simulink model "prova2"  (R2024a)
settings: Solver=ode23t  StartTime=0.0  StopTime=simT  RelTol=1e-3  AbsTol=1e-3
PreLoadFcn:
  | sscv_wind_turbine_input
undefined symbols (not defined in the file): actuatorRampRate, brakePressure, controllerTimeConstant, Derating, ee_sli_rtmsupport, G, gcbh, generatorEfficiency, generatorLumpedInductance, generatorLumpedResistance, gridFrequency, iGenerationGain, maxPitchAngle, minPitchAngle, mpptOmega, mpptPower, mpptWindSpeed, pGenerationGain, pGeneratorBrakeLimit, pitchBrakeAngle, turbineRatedPower, vWindRated, wAtGeneratorRatedPower, wGeneratorBrakeLimit
libraries: fl_lib x19, simulink x15, nesl_utility x14, ee_lib x10, sdl_lib x6, eeGeneralControl x3, eeGeneralMeasurement x2
(part 2 of 2)

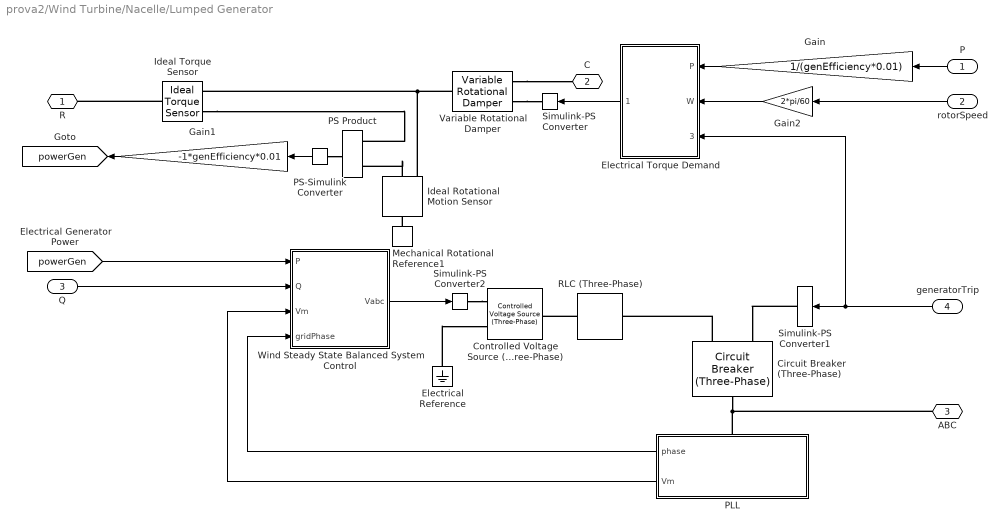
== system prova2/Wind Turbine/Nacelle/Lumped Generator ==
  P : Inport
  rotorSpeed : Inport  Port=2
  Q : Inport  Port=3
  generatorTrip : Inport  Port=4
  Circuit Breaker (Three-Phase) : ee_lib/Switches & Breakers/Circuit Breaker (Three-Phase)  R_closed=1e-5 Ohm  G_open=1e-8 1/Ohm  threshold=0.5 V  breaker_behavior=ee.enum.switches.breakerBehavior.zeroCrossingEnable
      settings: InternalSimscapePortConfiguration="{\"Bottom\":[],\"Left\":[{\"id\":\"vT\",\"label\":\"vT\",\"type\":\"input\"},{\"id\":\"N1\",\"label\":\"~1\",\"type\":\"foundation.electrical.three_phase\"}],\"Right\":[{\"id\":\"N2\",\"label\":\"~2\",\"type\":\"foundation.electrical.three_phase\"}],\"Top\":[]}"
  Controlled Voltage Source (Three-Phase) : ee_lib/Sources/Controlled Voltage Source (Three-Phase)  input_option=ee.enum.inputType.instantaneous  FRated=60 Hz
      settings: InternalSimscapePortConfiguration="{\"Bottom\":[],\"Left\":[{\"id\":\"S\",\"label\":\"S\",\"type\":\"input\"},{\"id\":\"n\",\"label\":\"n\",\"type\":\"foundation.electrical.electrical\"}],\"Right\":[{\"id\":\"N\",\"label\":\"~\",\"type\":\"foundation.electrical.three_phase\"}],\"Top\":[]}"
  Electrical Reference : fl_lib/Electrical/Electrical Elements/Electrical Reference
  Electrical Torque Demand : Subsystem
  Gain : Gain  Gain=1/(genEfficiency*0.01)
  Gain1 : Gain  Gain=-1*genEfficiency*0.01
  Gain2 : Gain  Gain=2*pi/60
  Ideal Rotational Motion Sensor : fl_lib/Mechanical/Mechanical Sensors/Ideal Rotational Motion Sensor  reference=foundation.enum.MeasurementReference.difference  acceleration_port=false  velocity_port=true  position_port=true  wrap_angle=simscape.enum.onoff.off  offset=0 rad
  Ideal Torque Sensor : fl_lib/Mechanical/Mechanical Sensors/Ideal Torque Sensor
  Mechanical Rotational Reference1 : fl_lib/Mechanical/Rotational Elements/Mechanical Rotational Reference
  PLL : Subsystem
      settings: PortSchema="{\"entries\":[{\"content\":{\"sides\":[{\"content\":{\"connectorIds\":[\"LConn1\"]},\"type\":\"ConnectorPlacement.EquallySpacedRectSide\",\"uuid\":\"d52864e1-db35-4dad-add5-1ee067043f1c\"},{\"content\":{\"connectorIds\":[],\"side\":\"RIGHT\"},\"type\":\"ConnectorPlacement.EquallySpacedRectSide\",\"uuid\":\"a5ba0e67-56ea-44cb-9ec3-4038d29660fe\"},{\"content\":{\"connectorIds\":[],\"side\":\"TOP\"},\"type\":\"ConnectorPlacement.EquallySpacedRectSide\",\"uuid\":\"5a398043-7e81-49e7-beae-eacc9cf31df4\"},{\"content\":{\"connectorIds\":[\"Out1\",\"Out2\"],\"side\":\"BOTTOM\"},\"type\":\"ConnectorPlacement.EquallySpacedRectSide\",\"uuid\":\"36c29948-68bf-4126-b9d0-685ba9cc8aca\"}]},\"type\":\"ConnectorPlacement.EquallySpacedConnector\",\"uuid\":\"348acdbb-59d7-41c8-861d-aa801afd2b04\"}],\"packageUris\":[\"http://schema.mathworks.com/mf0/Connector/R2020b\"],\"version\":\"1.0\"}"
  PS Product : fl_lib/Physical Signals/Functions/PS Product
  PS-Simulink Converter : nesl_utility/PS-Simulink Converter  PhysicalDomain=network_engine_domain  SubClassName=ps_output  LeftPortType=input  RightPortType=output  PseudoPeriodic=off  Frequencies=[]  VectorFormat=inherit  Unit=inherit  AffineConversion=off
  RLC (Three-Phase) : ee_lib/Passive/RLC Assemblies/RLC (Three-Phase)  component_structure=ee.enum.rlc.structure.SeriesRL  R=genResistor Ohm  L=genInductance H  C=1e-6 F  R_parasitic=0 Ohm  G_parasitic=0 1/Ohm  IL_specify=off  IL_priority=High  IL=[0, 0, 0] A  IL_nominal_specify=off  IL_nominal_value=1  IL_nominal_unit=A  VC_specify=off  VC_priority=High  VC=[0, 0, 0] V  VC_nominal_specify=off  VC_nominal_value=1  VC_nominal_unit=V
      settings: InternalSimscapePortConfiguration="{\"Bottom\":[],\"Left\":[{\"id\":\"N1\",\"label\":\"~1\",\"type\":\"foundation.electrical.three_phase\"}],\"Right\":[{\"id\":\"N2\",\"label\":\"~2\",\"type\":\"foundation.electrical.three_phase\"}],\"Top\":[]}"
  Simulink-PS Converter : nesl_utility/Simulink-PS Converter  PhysicalDomain=network_engine_domain  SubClassName=ps_input  LeftPortType=input  RightPortType=output  PseudoPeriodic=off  Frequencies=[]  NoiseDistribution=none  NoiseParameters=[]  Unit=N*m/(rad/s)  AffineConversion=off  FilteringAndDerivatives=provide  SimscapeFilterOrder=1  InputFilterTimeConstant=0.001  UdotUserProvided=0
  Simulink-PS Converter1 : nesl_utility/Simulink-PS Converter  PhysicalDomain=network_engine_domain  SubClassName=ps_input  LeftPortType=input  RightPortType=output  PseudoPeriodic=off  Frequencies=[]  NoiseDistribution=none  NoiseParameters=[]  Unit=V  AffineConversion=off  FilteringAndDerivatives=provide  SimscapeFilterOrder=1  InputFilterTimeConstant=0.001  UdotUserProvided=0
  Simulink-PS Converter2 : nesl_utility/Simulink-PS Converter  PhysicalDomain=network_engine_domain  SubClassName=ps_input  LeftPortType=input  RightPortType=output  PseudoPeriodic=off  Frequencies=[]  NoiseDistribution=none  NoiseParameters=[]  Unit=V  AffineConversion=off  FilteringAndDerivatives=provide  SimscapeFilterOrder=1  InputFilterTimeConstant=0.001  UdotUserProvided=0
  Variable Rotational Damper : sdl_lib/Couplings & Drives/Springs & Dampers/Variable Rotational Damper  Bmin=1e-3 N*m*s/rad
      settings: InternalSimscapePortConfiguration="{\"Bottom\":[],\"Left\":[{\"id\":\"B\",\"label\":\"B\",\"type\":\"input\"},{\"id\":\"R\",\"label\":\"R\",\"type\":\"foundation.mechanical.rotational.rotational\"}],\"Right\":[{\"id\":\"C\",\"label\":\"C\",\"type\":\"foundation.mechanical.rotational.rotational\"}],\"Top\":[]}"
  Wind Steady State Balanced System Control : Subsystem
  R : PMIOPort  Side=Left
  C : PMIOPort  Port=2  Side=Left
  ABC : PMIOPort  Port=3  Side=Right
  tag scope: powerGen=global
  wires:
  Wind Steady State Balanced System Control/1(Vabc) -> Simulink-PS Converter2/1
  Q/1 -> Wind Steady State Balanced System Control/2(Q)
  P/1 -> Gain/1
  rotorSpeed/1 -> Gain2/1
  PS-Simulink Converter/1 -> Gain1/1
  PLL/1(phase) -> Wind Steady State Balanced System Control/4(gridPhase)
  Electrical Torque Demand/1(Damping) -> Simulink-PS Converter/1
  Gain2/1 -> Electrical Torque Demand/2(W)
  Gain/1 -> Electrical Torque Demand/1(P)
  Gain1/1 -> [powerGen]
  [powerGen] -> Wind Steady State Balanced System Control/1(P)
  PLL/2(Vm) -> Wind Steady State Balanced System Control/3(Vm)
  generatorTrip/1 -> Simulink-PS Converter1/1, Electrical Torque Demand/3(generatorTrip)
  connections:
  RLC (Three-Phase)/LConn1 -- Controlled Voltage Source (Three-Phase)/RConn1
  Ideal Rotational Motion Sensor/RConn1 -- Variable Rotational Damper/RConn1 -- Ideal Torque Sensor/RConn1
  Ideal Torque Sensor/LConn1 -- R/RConn1
  Ideal Torque Sensor/RConn2 -- PS Product/LConn2
  Mechanical Rotational Reference1/LConn1 -- Ideal Rotational Motion Sensor/LConn1
  Simulink-PS Converter2/RConn1 -- Controlled Voltage Source (Three-Phase)/LConn1
  Electrical Reference/LConn1 -- Controlled Voltage Source (Three-Phase)/LConn2
  Ideal Rotational Motion Sensor/RConn2 -- PS Product/LConn1
  PS-Simulink Converter/LConn1 -- PS Product/RConn1
  Circuit Breaker (Three-Phase)/RConn1 -- ABC/RConn1 -- PLL/LConn1
  Circuit Breaker (Three-Phase)/LConn2 -- RLC (Three-Phase)/RConn1
  Simulink-PS Converter1/RConn1 -- Circuit Breaker (Three-Phase)/LConn1
  Variable Rotational Damper/LConn1 -- Simulink-PS Converter/RConn1
  Variable Rotational Damper/LConn2 -- C/RConn1

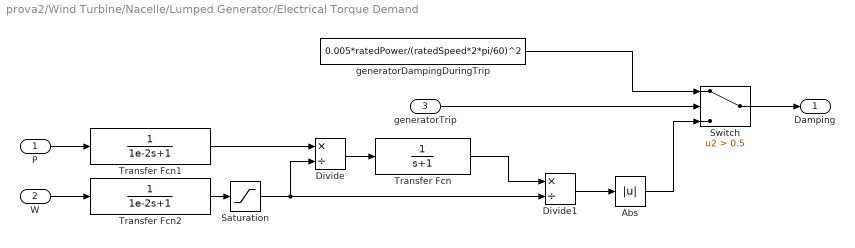
== system prova2/Wind Turbine/Nacelle/Lumped Generator/Electrical Torque Demand ==
  P : Inport
  W : Inport  Port=2
  generatorTrip : Inport  Port=3
  Abs : Abs  SaturateOnIntegerOverflow=off
  Divide : Product  Inputs=*/
  Divide1 : Product  Inputs=*/
  Saturation : Saturate  UpperLimit=inf  LowerLimit=0.2*ratedSpeed*2*pi/60
  Switch : Switch  Criteria=u2 > Threshold  Threshold=0.5  SaturateOnIntegerOverflow=off  InputSameDT=off
  Transfer Fcn : TransferFcn  Denominator=[1 1]
  Transfer Fcn1 : TransferFcn  Denominator=[1e-2 1]
  Transfer Fcn2 : TransferFcn  Denominator=[1e-2 1]
  generatorDampingDuringTrip : Constant  Value=0.005*ratedPower/(ratedSpeed*2*pi/60)^2
  Damping : Outport
  wires:
  Divide1/1 -> Abs/1
  Divide/1 -> Transfer Fcn/1
  Transfer Fcn/1 -> Divide1/1
  W/1 -> Transfer Fcn2/1
  Transfer Fcn1/1 -> Divide/1
  P/1 -> Transfer Fcn1/1
  Transfer Fcn2/1 -> Saturation/1
  Saturation/1 -> Divide1/2, Divide/2
  generatorTrip/1 -> Switch/2
  Abs/1 -> Switch/3
  Switch/1 -> Damping/1
  generatorDampingDuringTrip/1 -> Switch/1

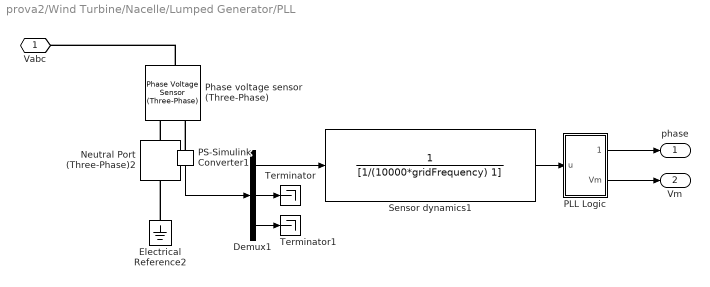
== system prova2/Wind Turbine/Nacelle/Lumped Generator/PLL ==
  Demux1 : Demux  Outputs=3
  Electrical Reference2 : fl_lib/Electrical/Electrical Elements/Electrical Reference
  Neutral Port (Three-Phase)2 : ee_lib/Connectors & References/Neutral Port (Three-Phase)  G_parasitic=1e-12 1/Ohm
      settings: InternalSimscapePortConfiguration="{\"Bottom\":[],\"Left\":[{\"id\":\"N\",\"label\":\"~\",\"type\":\"foundation.electrical.three_phase\"}],\"Right\":[{\"id\":\"n\",\"label\":\"n\",\"type\":\"foundation.electrical.electrical\"}],\"Top\":[]}"
  PLL Logic : Subsystem
  PS-Simulink Converter1 : nesl_utility/PS-Simulink Converter  PhysicalDomain=network_engine_domain  SubClassName=ps_output  LeftPortType=input  RightPortType=output  PseudoPeriodic=off  Frequencies=[]  VectorFormat=1-D array  Unit=inherit  AffineConversion=off
  Phase voltage sensor (Three-Phase) : ee_lib/Sensors & Transducers/Phase Voltage Sensor (Three-Phase)
  Sensor dynamics1 : TransferFcn  Numerator=1  Denominator=[1/(10000*gridFrequency) 1]
  Terminator : Terminator
  Terminator1 : Terminator
  Vabc : PMIOPort  Side=Left
  phase : Outport
  Vm : Outport  Port=2
  wires:
  Demux1/3 -> Terminator1/1
  PLL Logic/1(phase) -> phase/1
  Sensor dynamics1/1 -> PLL Logic/1(u)
  PS-Simulink Converter1/1 -> Demux1/1
  Demux1/1 -> Sensor dynamics1/1
  Demux1/2 -> Terminator/1
  PLL Logic/2(Vm) -> Vm/1
  connections:
  PS-Simulink Converter1/LConn1 -- Phase voltage sensor (Three-Phase)/RConn1
  Neutral Port (Three-Phase)2/LConn1 -- Phase voltage sensor (Three-Phase)/RConn2
  Electrical Reference2/LConn1 -- Neutral Port (Three-Phase)2/RConn1
  Phase voltage sensor (Three-Phase)/LConn1 -- Vabc/RConn1

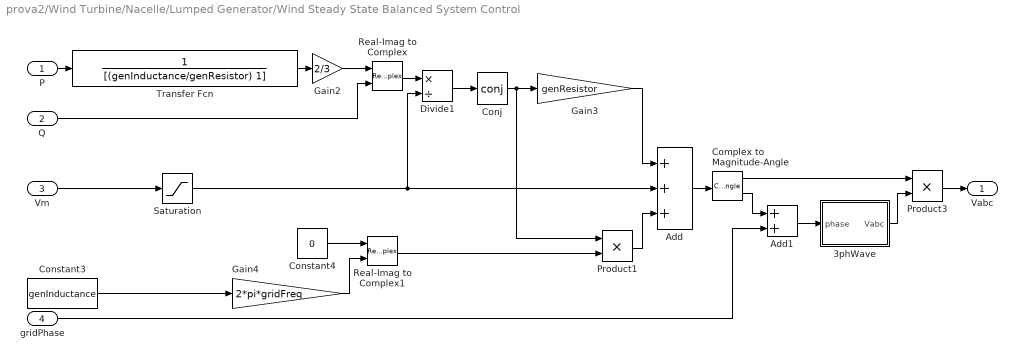
== system prova2/Wind Turbine/Nacelle/Lumped Generator/Wind Steady State Balanced System Control ==
  P : Inport
  Q : Inport  Port=2
  Vm : Inport  Port=3
  gridPhase : Inport  Port=4
  3phWave : Subsystem
  Add : Sum  Inputs=+++
  Add1 : Sum
  Complex to Magnitude-Angle : ComplexToMagnitudeAngle
  Conj : Math  Operator=conj
  Constant3 : Constant  Value=genInductance
  Constant4 : Constant  Value=0
  Divide1 : Product  Inputs=*/
  Gain2 : Gain  Gain=2/3
  Gain3 : Gain  Gain=genResistor
  Gain4 : Gain  Gain=2*pi*gridFreq
  Product1 : Product
  Product3 : Product
  Real-Imag to Complex : RealImagToComplex
  Real-Imag to Complex1 : RealImagToComplex
  Saturation : Saturate  UpperLimit=10000  LowerLimit=10
  Transfer Fcn : TransferFcn  Denominator=[(genInductance/genResistor) 1]
  Vabc : Outport
  wires:
  Add1/1 -> 3phWave/1(phase)
  Divide1/1 -> Conj/1
  Complex to Magnitude-Angle/2 -> Add1/1
  3phWave/1(Vabc) -> Product3/2
  Complex to Magnitude-Angle/1 -> Product3/1
  Gain4/1 -> Real-Imag to Complex1/2
  Gain3/1 -> Add/1
  Add/1 -> Complex to Magnitude-Angle/1
  Real-Imag to Complex/1 -> Divide1/1
  Constant3/1 -> Gain4/1
  Conj/1 -> Gain3/1, Product1/1
  Product3/1 -> Vabc/1
  Saturation/1 -> Add/2, Divide1/2
  Gain2/1 -> Real-Imag to Complex/1
  gridPhase/1 -> Add1/2
  Constant4/1 -> Real-Imag to Complex1/1
  Real-Imag to Complex1/1 -> Product1/2
  Vm/1 -> Saturation/1
  Product1/1 -> Add/3
  Q/1 -> Real-Imag to Complex/2
  Transfer Fcn/1 -> Gain2/1
  P/1 -> Transfer Fcn/1

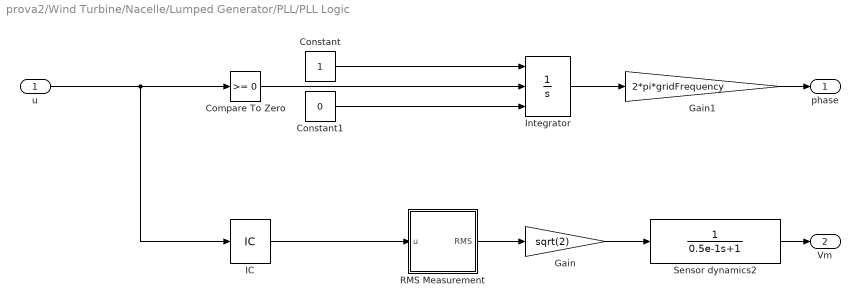
== system prova2/Wind Turbine/Nacelle/Lumped Generator/PLL/PLL Logic ==
  u : Inport
  Compare To Zero : simulink/Logic and Bit Operations/Compare To Zero  relop=>=  OutDataTypeStr=boolean
  Constant : Constant
  Constant1 : Constant  Value=0
  Gain : Gain  Gain=sqrt(2)
  Gain1 : Gain  Gain=2*pi*gridFrequency
  IC : InitialCondition  Value=1e-4
  Integrator : Integrator  ExternalReset=rising  InitialConditionSource=external  WrapState=on  WrappedStateUpperValue=pi*2  WrappedStateLowerValue=0
  RMS Measurement : Subsystem  LoadFcn=ee_sli_rtmsupport( 'loadfcn', gcbh );  Variant=on  VariantControlMode=label  LabelModeActiveChoice=Total  mask(RMS Measurement){F=gridFrequency, SpecifyHarmonics=off, K=[0 1 2], Ts=0}
      mask prompts: F "physmod:ee:library:comments:control:eeRmsMeasurement:BaseFrequencyHz_MP"; SpecifyHarmonics "physmod:ee:library:comments:control:eeRmsMeasurement:SpecifyHarmonics_MP"; K "physmod:ee:library:comments:control:eeRmsMeasurement:HarmonicNumbers_MP"; Ts "physmod:ee:library:comments:control:eeRmsMeasurement:SampleTime_MP"
      mask help: physmod:ee:library:comments:control:eeRmsMeasurement:RMSMeasurement_MD
      mask init:
      | [timeDomain,G]=ee.mask.initializeRmsMeasurement(gcb,F,Ts,K,SpecifyHarmonics);
      settings: CopyFcn=ee_sli_rtmsupport( 'copyfcn', gcbh );  DeleteFcn=ee_sli_rtmsupport( 'deletefcn', gcbh );  ModelCloseFcn=ee_sli_rtmsupport( 'modelclosefcn', gcbh );  PostSaveFcn=ee_sli_rtmsupport( 'postsavefcn', gcbh );  PreCopyFcn=ee_sli_rtmsupport( 'precopyfcn', gcbh );  OpenFcn=ee_sli_rtmsupport( 'openfcn', gcbh );  CloseFcn=ee_sli_rtmsupport( 'closefcn', gcbh );  PreDeleteFcn=ee_sli_rtmsupport( 'predeletefcn', gcbh );
      mask Help: web(nesl_help(gcbh))
      mask Callback SpecifyHarmonics: ee.mask.callbackRmsMeasurement(gcb);
      mask TypeOptions Ts:
      | Total RMS/Integrator
      | (Discrete or Continuous)/Ts | Total RMS/Periodic Difference
      | (Discrete or Continuous)/Ts | Harmonic RMS/Integrator
      | (Discrete or Continuous)/Ts | Harmonic RMS/SinCos/Integrator with
      | Wrapped State
      | (Discrete or Continuous)/Ts | Harmonic RMS/Periodic Difference
      | (Discrete or Continuous)/Ts
      mask DialogControl F Prompt: Base frequency (Hz)
      mask DialogControl SpecifyHarmonics Prompt: Specify harmonics
      mask DialogControl K Prompt: Harmonic numbers
      mask DialogControl Ts Prompt: Sample time
      mask Display: ee.mask.drawRmsMeasurement;
  Sensor dynamics2 : TransferFcn  Numerator=1  Denominator=[0.5e-1 1]
  phase : Outport
  Vm : Outport  Port=2
  wires:
  Integrator/1 -> Gain1/1
  Constant/1 -> Integrator/1
  Compare To Zero/1 -> Integrator/2
  Constant1/1 -> Integrator/3
  Gain1/1 -> phase/1
  RMS Measurement/1(RMS) -> Gain/1
  Gain/1 -> Sensor dynamics2/1
  IC/1 -> RMS Measurement/1(u)
  Sensor dynamics2/1 -> Vm/1
  u/1 -> IC/1, Compare To Zero/1

== system prova2/Wind Turbine/Nacelle/Lumped Generator/Wind Steady State Balanced System Control/3phWave ==
  phase : Inport
  Add Constant : Bias  Bias=-120*pi/180  SaturateOnIntegerOverflow=off
  Add Constant1 : Bias  Bias=120*pi/180  SaturateOnIntegerOverflow=off
  Mux : Mux  Inputs=3
  Trigonometric Function : Trigonometry
  Vabc : Outport
  wires:
  Mux/1 -> Trigonometric Function/1
  phase/1 -> Add Constant1/1, Add Constant/1, Mux/1
  Add Constant/1 -> Mux/2
  Add Constant1/1 -> Mux/3
  Trigonometric Function/1 -> Vabc/1

== system prova2/Wind Turbine/Nacelle/Lumped Generator/PLL/PLL Logic/RMS Measurement ==
  u : Inport
  Harmonic RMS : Subsystem  VariantControl=Harmonic
  Total RMS : Subsystem  VariantControl=Total
  RMS : Outport  VectorParamsAs1DForOutWhenUnconnected=off

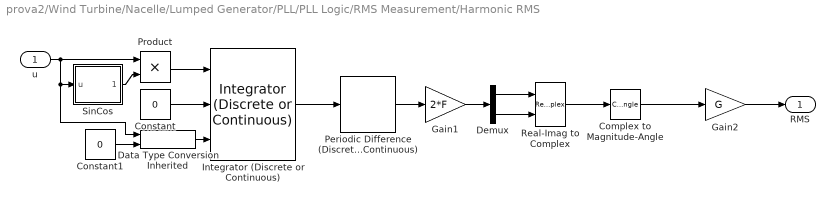
== system prova2/Wind Turbine/Nacelle/Lumped Generator/PLL/PLL Logic/RMS Measurement/Harmonic RMS ==
  u : Inport
  Complex to Magnitude-Angle : ComplexToMagnitudeAngle  Output=Magnitude
  Constant : Constant  Value=0
  Constant1 : Constant  Value=0
  Data Type Conversion Inherited : simulink/Signal Attributes/Data Type Conversion Inherited  ConvertRealWorld=Real World Value  DoSatur=off
  Demux : Demux  Outputs=2
  Gain1 : Gain  Gain=2*F
  Gain2 : Gain  Gain=G
  Integrator (Discrete or Continuous) : eeGeneralControl/Integrator (Discrete or Continuous)  LabelModeActiveChoice=Continuous  ExternalReset=level  LimitType=Anti-windup  B=inf  A=-inf  Ts=Ts
  Periodic Difference (Discrete or Continuous) : eeGeneralMeasurement/Periodic Difference (Discrete or Continuous)  LabelModeActiveChoice=Continuous  F=F  Ts=Ts
  Product : Product
  Real-Imag to Complex : RealImagToComplex
  SinCos : Subsystem
  RMS : Outport  VectorParamsAs1DForOutWhenUnconnected=off
  wires:
  Constant1/1 -> Data Type Conversion Inherited/2
  Data Type Conversion Inherited/1 -> Integrator (Discrete or Continuous)/3
  Integrator (Discrete or Continuous)/1 -> Periodic Difference (Discrete or Continuous)/1
  Constant/1 -> Integrator (Discrete or Continuous)/2
  Gain2/1 -> RMS/1
  Demux/2 -> Real-Imag to Complex/2
  u/1 -> SinCos/1(u), Data Type Conversion Inherited/1, Product/1
  Periodic Difference (Discrete or Continuous)/1 -> Gain1/1
  Real-Imag to Complex/1 -> Complex to Magnitude-Angle/1
  Demux/1 -> Real-Imag to Complex/1
  SinCos/1(SinCos) -> Product/2
  Gain1/1 -> Demux/1
  Product/1 -> Integrator (Discrete or Continuous)/1
  Complex to Magnitude-Angle/1 -> Gain2/1

== system prova2/Wind Turbine/Nacelle/Lumped Generator/PLL/PLL Logic/RMS Measurement/Total RMS ==
  u : Inport
  Abs : Abs  SaturateOnIntegerOverflow=off
  Constant : Constant  Value=0
  Constant1 : Constant  Value=0
  Data Type Conversion Inherited : simulink/Signal Attributes/Data Type Conversion Inherited  ConvertRealWorld=Real World Value  DoSatur=off
  Gain : Gain  Gain=F
  Integrator (Discrete or Continuous) : eeGeneralControl/Integrator (Discrete or Continuous)  LabelModeActiveChoice=Continuous  ExternalReset=level  LimitType=Anti-windup  B=inf  A=-inf  Ts=Ts
  Math Function : Math  Operator=square  SignedPower=on
  Periodic Difference (Discrete or Continuous) : eeGeneralMeasurement/Periodic Difference (Discrete or Continuous)  LabelModeActiveChoice=Continuous  F=F  Ts=Ts
  Sqrt : Sqrt
  RMS : Outport  VectorParamsAs1DForOutWhenUnconnected=off
  wires:
  Constant1/1 -> Data Type Conversion Inherited/2
  Data Type Conversion Inherited/1 -> Integrator (Discrete or Continuous)/3
  Periodic Difference (Discrete or Continuous)/1 -> Gain/1
  Sqrt/1 -> RMS/1
  Integrator (Discrete or Continuous)/1 -> Periodic Difference (Discrete or Continuous)/1
  u/1 -> Math Function/1
  Math Function/1 -> Integrator (Discrete or Continuous)/1, Data Type Conversion Inherited/1
  Constant/1 -> Integrator (Discrete or Continuous)/2
  Gain/1 -> Abs/1
  Abs/1 -> Sqrt/1

== system prova2/Wind Turbine/Nacelle/Lumped Generator/PLL/PLL Logic/RMS Measurement/Harmonic RMS/SinCos ==
  u : Inport
  Data Type Conversion Inherited : simulink/Signal Attributes/Data Type Conversion Inherited  ConvertRealWorld=Real World Value  DoSatur=off
  Integrator with Wrapped State (Discrete or Continuous) : eeGeneralControl/Integrator with Wrapped State (Discrete or Continuous)  LabelModeActiveChoice=Continuous  WrappedStateUpperValue=2*pi  WrappedStateLowerValue=0  x0=0  Ts=Ts
  Mux : Mux  Inputs=2
  Radial frequencies : Constant  Value=2*pi*F*K
  sincos : Trigonometry  Operator=sincos
  SinCos : Outport  VectorParamsAs1DForOutWhenUnconnected=off
  wires:
  u/1 -> Data Type Conversion Inherited/1
  Radial frequencies/1 -> Data Type Conversion Inherited/2
  Data Type Conversion Inherited/1 -> Integrator with Wrapped State (Discrete or Continuous)/1
  Integrator with Wrapped State (Discrete or Continuous)/1 -> sincos/1
  Mux/1 -> SinCos/1
  sincos/1 -> Mux/1
  sincos/2 -> Mux/2

== stateflow chart prova2/Turbine State Machine ==
  state Startup
    entry: parkingBrake = 0;
    generatorTrip = 1;
    pitchBrake = 0;
    turbineState = 1;
  state Generating
    entry: parkingBrake = 0;
    generatorTrip = 0;
    pitchBrake = 0;
    turbineState = 2;
  state ParkBrake
    entry: parkingBrake = 1;
    generatorTrip = 1;
    pitchBrake = 1;
    turbineState = 0;
  state PitchBrake
    entry: parkingBrake = 0;
    generatorTrip = 0;
    pitchBrake = 1;
    turbineState = 3;
  (junction 37) -> Startup : [duration(windSpeed>...
      | wind_speed_cut_in_lower)>0.10...
      | &&duration(windSpeed<...
      | wind_speed_cut_out)>0.10]
  ParkBrake -> (junction 37)
  Startup -> (junction 41) [order 1] : [duration(turbineSpeed>...
      | turbine_speed_cut_in)>0.10]
  (junction 41) -> Generating
  Startup -> PitchBrake [order 2] : [duration(windSpeed<...
      | wind_speed_cut_in_lower)>1.0...
      | ||duration(windSpeed>...
      | wind_speed_cut_out)>1.0]
  PitchBrake -> Startup [order 2] : [duration(windSpeed<=...
      | wind_speed_cut_in_upper)>2.0...
      | && duration(windSpeed>...
      | wind_speed_cut_in_lower)>2.0...
      | && duration(turbineSpeed<...
      | turbine_speed_cut_in)>2.0]
  (default) -> ParkBrake
  Generating -> (junction 43) : [duration(windSpeed<...
      | wind_speed_cut_in_lower)>0.10...
      | ||duration(windSpeed>...
      | wind_speed_cut_out)>0.10...
      | ||duration(turbineSpeed>...
      | turbine_speed_cut_out)>0.10...
      | ||duration(turbineSpeed<...
      | turbine_speed_cut_in)>0.10]
  (junction 39) -> ParkBrake
  PitchBrake -> (junction 39) [order 1] : [duration(turbineSpeed<=...
      | park_speed)>0.10]
  (junction 43) -> PitchBrake
  data: pitchBrake output double; windSpeed input; turbineSpeed input; parkingBrake output double; generatorTrip output double; wind_speed_cut_in_lower local double =vWindCutInLower; turbine_speed_cut_in local double =wTurbineCutIn; turbineState output double; wind_speed_cut_out local double =vWindCutOut; wind_speed_cut_in_upper local double =vWindCutInUpper; turbine_speed_cut_out local double =wTurbineCutOut; park_speed constant double =wTurbinePark
